simulink model "A3_PID_A_AttitudeDynamics"  (R2017b)
settings: Solver=VariableStepAuto  StartTime=0.0  StopTime=20  FixedStep=1  MaxStep=0.1  RelTol=1e-6  EnableMultiTasking=on
PostLoadFcn:
  | AttitudeDynamicsData;
StopFcn:
  | attitudePlot = animateAttitude(rotmOut, 0.016);
  | attitudePlot.plotInit;
  | responsePlot(responseData, rotmOut, omegaRsOut, mechEnergyOut, mechPowerOut, torqueOut);
values from neighbouring files (symbols this model uses):
  J_sat = [2.5 2.5 2.5]    [AttitudeDynamicsData.m]
  PID_A = struct(      'P', 0.4,          'I', 0.01,     'D', 3          )    [AttitudeDynamicsData.m]
  T_disturb = ones(1,3) * 0.1E-3    [AttitudeDynamicsData.m]
undefined symbols (not defined in the file or in its folder): DiscIntNeverNeededParam
libraries: SatelliteLibrary x14
(part 2 of 2)

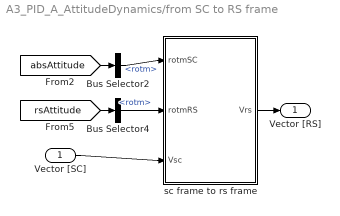
== system A3_PID_A_AttitudeDynamics/from SC to RS frame ==
  Vector [SC] : Inport
  Bus Selector2 : BusSelector  OutputSignals=rotm
  Bus Selector4 : BusSelector  OutputSignals=rotm
  sc frame to rs frame : MATLAB Function  TreatAsAtomicUnit=on
  Vector [RS] : Outport
  wires:
  Vector [SC]/1 -> sc frame to rs frame/3(Vsc)
  sc frame to rs frame/1(Vrs) -> Vector [RS]/1
  [rsAttitude] -> Bus Selector4/1
  Bus Selector4/1 -> sc frame to rs frame/2(rotmRS)  "<rotm>"
  [absAttitude] -> Bus Selector2/1
  Bus Selector2/1 -> sc frame to rs frame/1(rotmSC)  "<rotm>"

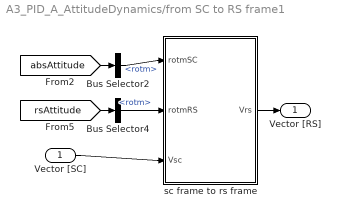
== system A3_PID_A_AttitudeDynamics/from SC to RS frame1 ==
  Vector [SC] : Inport
  Bus Selector2 : BusSelector  OutputSignals=rotm
  Bus Selector4 : BusSelector  OutputSignals=rotm
  sc frame to rs frame : MATLAB Function  TreatAsAtomicUnit=on
  Vector [RS] : Outport
  wires:
  Vector [SC]/1 -> sc frame to rs frame/3(Vsc)
  sc frame to rs frame/1(Vrs) -> Vector [RS]/1
  [rsAttitude] -> Bus Selector4/1
  Bus Selector4/1 -> sc frame to rs frame/2(rotmRS)  "<rotm>"
  [absAttitude] -> Bus Selector2/1
  Bus Selector2/1 -> sc frame to rs frame/1(rotmSC)  "<rotm>"

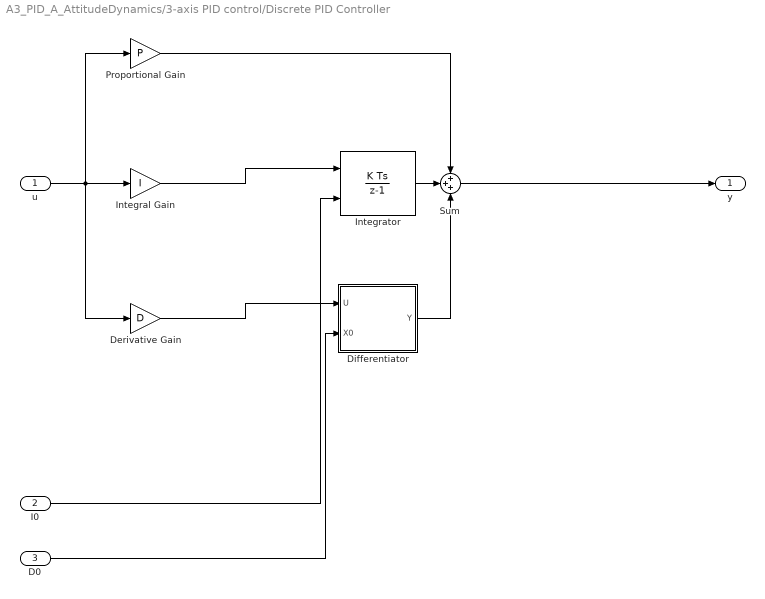
== system A3_PID_A_AttitudeDynamics/3-axis PID control/Discrete PID Controller ==
  u : Inport  SampleTime=SampleTime
  I0 : Inport  Port=2  SampleTime=SampleTime
  D0 : Inport  Port=3  SampleTime=SampleTime
  Derivative Gain : Gain  DisableCoverage=on  Gain=D  ParamMin=DParamMin  ParamMax=DParamMax  OutMin=DOutMin  OutMax=DOutMax  SampleTime=SampleTime
  Differentiator : Subsystem
      mask Display: text(0.5, 0.5, '(z-1)', 'horizontalAlignment', 'center', 'verticalAlignment', 'bottom');text(0.5, 0.5, 'Ts z', 'horizontalAlignment', 'center', 'verticalAlignment', 'top');plot([0.3 0.7],[0.5 0.5]);port_label('input', 2, '\rmx_0', 'texmode', 'on');
  Integral Gain : Gain  DisableCoverage=on  Gain=I  ParamMin=IParamMin  ParamMax=IParamMax  OutMin=IOutMin  OutMax=IOutMax  SampleTime=SampleTime
  Integrator : DiscreteIntegrator  InitialConditionSource=external  InitialCondition=InitialConditionForIntegrator  InitialConditionSetting=State (most efficient)  SampleTime=SampleTime  OutMin=IntegratorOutMin  OutMax=IntegratorOutMax  ICPrevOutput=DiscIntNeverNeededParam  ICPrevScaledInput=DiscIntNeverNeededParam
  Proportional Gain : Gain  Gain=P  ParamMin=PParamMin  ParamMax=PParamMax  OutMin=POutMin  OutMax=POutMax  SampleTime=SampleTime
  Sum : Sum  Inputs=+++  OutMin=SumOutMin  OutMax=SumOutMax  SampleTime=SampleTime
  y : Outport  SampleTime=SampleTime  InitialOutput=0
  wires:
  u/1 -> Integral Gain/1, Derivative Gain/1, Proportional Gain/1
  Integral Gain/1 -> Integrator/1
  Integrator/1 -> Sum/2
  Derivative Gain/1 -> Differentiator/1(U)
  Differentiator/1(Y) -> Sum/3
  Proportional Gain/1 -> Sum/1
  Sum/1 -> y/1
  I0/1 -> Integrator/2
  D0/1 -> Differentiator/2(X0)

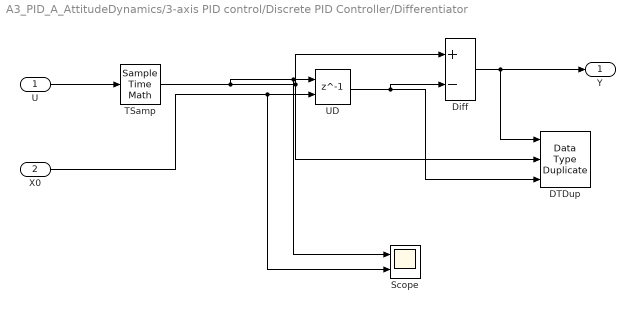
== system A3_PID_A_AttitudeDynamics/3-axis PID control/Discrete PID Controller/Differentiator ==
  U : Inport  SampleTime=SampleTime
  X0 : Inport  Port=2
  DTDup : DataTypeDuplicate  NumInputPorts=3
  Diff : Sum  Inputs=+-  OutMin=DifferentiatorOutMin  OutMax=DifferentiatorOutMax  OutDataTypeStr=Inherit: Inherit via back propagation  InputSameDT=on
  Scope : Scope  NumInputPorts=2
  TSamp : SampleTimeMath  TsampMathOp=/  TsampMathImp=Offline Scaling Adjustment
  UD : Delay  DelayLength=1  InitialConditionSource=Input port  InitialCondition=DifferentiatorICPrevScaledInput  InputProcessing=Inherited
      settings: InputPortMap=u0,p4
  Y : Outport  OutMin=DifferentiatorOutMin  OutMax=DifferentiatorOutMax  SampleTime=SampleTime
  wires:
  U/1 -> TSamp/1
  TSamp/1 -> Diff/1, DTDup/2, Scope/1, UD/1
  UD/1 -> Diff/2, DTDup/3
  Diff/1 -> Y/1, DTDup/1
  X0/1 -> Scope/2, UD/2

== matlab function A3_PID_A_AttitudeDynamics/Calculate Relative Attitude/minimum rotation quaternion ==
  data: q input; qPos output
function qPos = minRotation(q)
    % converts quaternion to form of smalest angle (last element always <0, 1] )
    if q(4) < 0
        qPos = -q;
    else
        qPos = q;
    end
end

== matlab function A3_PID_A_AttitudeDynamics/from SC to RS frame/sc frame to rs frame ==
  data: rotmSC input; Vrs output; rotmRS input; Vsc input
function ...
    Vrs               ...
  = sc2rs(            ...
    rotmSC,         ...
    rotmRS,         ...
    Vsc             ...
    )
    % transform vector in spacecraft (SC) frame into vector in
    % reactionsphere (RS) frame.
    Vrs = rotmRS' * rotmSC * Vsc;

end

== matlab function A3_PID_A_AttitudeDynamics/Calculate Relative Attitude/relative rotation matrix ==
  data: CAbs input; COrb input; CRel output
function CRel = rotmatRelative(...
    CAbs, ... absolute rotation matrix orientation (in inertial reference frame)
    COrb  ... orbital frame rotation matrix orientation
    )

CRel = COrb' * CAbs;
end

== matlab function A3_PID_A_AttitudeDynamics/Axis Angle Error/minimum rotation quaternion ==
  data: q input; qPos output
function qPos = minRotation(q)
    % converts quaternion to form of smalest angle (last element always <0, 1] )
    if q(4) < 0
        qPos = -q;
    else
        qPos = q;
    end
end

== matlab function A3_PID_A_AttitudeDynamics/Calculate Relative Attitude/relative quaternion ==
  data: qA input; qO input; qRel output
function qRel = quatRelative(...
    qA, ... absolute quaternion orientation (in inertial reference frame)
    qO  ... orbital frame quaternion orientation
    )
% Calculate the error quaternion
% q_... are standard quaternions with the vector part at the start

qOinv = [-qO(1:3); qO(4)];
qAmatrix = [ qA(4)  qA(3) -qA(2)  qA(1);...
            -qA(3)  qA(4)  qA(1)  qA(2);...
             qA(2) -qA(1)  qA(4)  qA(3);...
            -qA(1) -qA(2) -qA(3)  qA(4)];
qRel = qAmatrix * qOinv;
end

== matlab function A3_PID_A_AttitudeDynamics/from SC to RS frame1/sc frame to rs frame ==
  data: rotmSC input; Vrs output; rotmRS input; Vsc input
function ...
    Vrs               ...
  = sc2rs(            ...
    rotmSC,         ...
    rotmRS,         ...
    Vsc             ...
    )
    % transform vector in spacecraft (SC) frame into vector in
    % reactionsphere (RS) frame.
    Vrs = rotmRS' * rotmSC * Vsc;

end
